simulink model "rlgrindingsystemPIDTune"  (R2024b)
settings: Solver=ode45  StartTime=0.0  StopTime=200  RelTol=1e-3  EnableMultiTasking=on
undefined symbols (not defined in the file or in its folder): DiscIntNeverNeededParam, Ts
libraries: rllib x1
settings Model: Creator=The MathWorks, Inc.  LastModifiedBy=phama
settings SolverCC: AlgebraicLoopSolver=TrustRegion  MaxZcPerStep=1
settings DataIOCC: LimitDataPoints=on  SaveFormat=Array  SignalLoggingName=logsOut
settings OptimizationCC: ExpressionDepthLimit=2147483647  InitFltsAndDblsToZero=on  LifeSpan=inf
settings DebuggingCC: SaveWithParameterizedLinksMsg=none  UnderspecifiedInitializationDetection=Classic  MergeDetectMultiDrivingBlocksExec=none  SignalResolutionControl=TryResolveAllWithWarning  MultiTaskDSMMsg=warning  FcnCallInpInsideContextMsg=warning  UnconnectedInputMsg=warning  UnconnectedOutputMsg=warning  UnconnectedLineMsg=warning  AllowSymbolicDim=off  StateNameClashWarn=warning  SFUnexpectedBacktrackingDiag=warning  SFNoUnconditionalDefaultTransitionDiag=warning  SFExecutionAtInitializationDiag=none  ArithmeticOperatorsInVariantConditions=warning
settings HardwareCC: ProdBitPerPointer=32  ProdBitPerSizeT=32  ProdBitPerPtrDiffT=32  ProdLargestAtomicFloat=None  ProdIntDivRoundTo=Undefined  ProdEndianess=Unspecified  ProdWordSize=32  ProdHWDeviceType=Specified
settings ModelReferenceCC: EnableRefExpFcnMdlSchedulingChecks=on  PropagateSignalLabelsOutOfModel=off
settings SFSimCC: SimUseLocalCustomCode=off
settings RTWCC: RTWUseLocalCustomCode=off  GPUComputeCapability=3.5  DLArmComputeVersion=19.05
settings CodeAppCC: StateflowObjectComments=on
settings GRTTargetCC: TargetFcnLib=ansi_tfl_tmw.mat  TargetLangStandard=C89/C90 (ANSI)  CombineOutputUpdateFcns=off  GRTInterface=on
settings ConfigComp: CovMetricSettings=dw  CovSaveCumulativeToWorkspaceVar=on  CovSaveSingleToWorkspaceVar=on  CovExternalEMLEnable=off

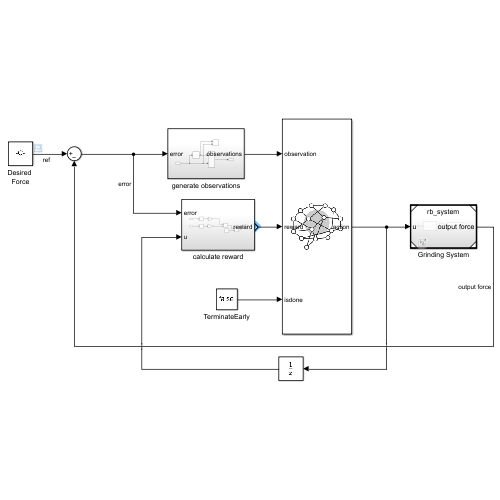
[thumbnail: Simulink's stored preview of the top-level diagram]
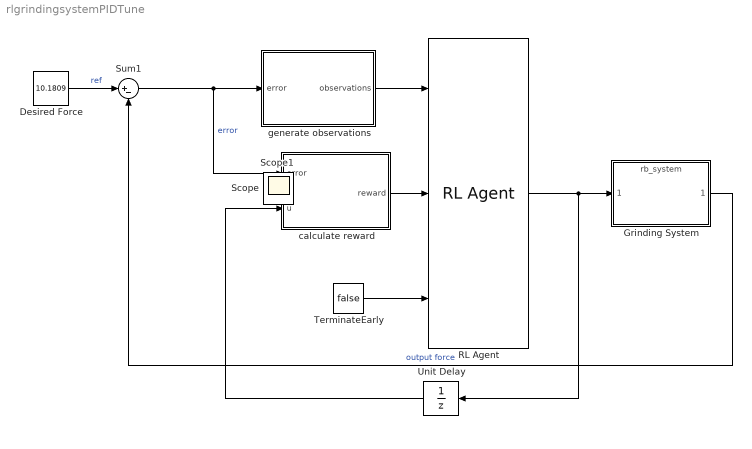
== system rlgrindingsystemPIDTune ==
  Desired Force : Constant  Value=10.1809
  Grinding System : ModelReference  ModelNameDialog=rb_system.slx  SimulationMode=Normal  ModelReferenceVersion=1.5
  RL Agent : rllib/RL Agent  Agent=agent  ExternalActionAsInput=off  ProvideLastAction=off  ProvideCumRwd=off  TreatAsDirectFeedthrough=on  UseStrictObservationDataTypes=off
  Sum1 : Sum  Inputs=|+-  SaturateOnIntegerOverflow=on
  TerminateEarly : Constant  Value=false
  Unit Delay : UnitDelay  SampleTime=-1  HasFrameUpgradeWarning=on
  calculate reward : Subsystem
  generate observations : Subsystem
  Scope : Scope
  Scope1 : Scope
  wires:
  Desired Force/1 -> Sum1/1  "ref"
  Sum1/1 -> calculate reward/1(error), generate observations/1(error)  "error"
  generate observations/1(observations) -> RL Agent/1
  RL Agent/1 -> Grinding System/1, Unit Delay/1
  Grinding System/1 -> Sum1/2  "output force"
  Unit Delay/1 -> calculate reward/2(u)
  calculate reward/1(reward) -> RL Agent/2
  TerminateEarly/1 -> RL Agent/3

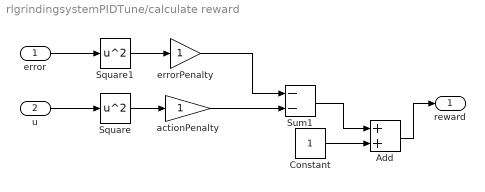
== system rlgrindingsystemPIDTune/calculate reward ==
  error : Inport
  u : Inport  Port=2
  Add : Sum
  Constant : Constant
  Square : Math  Operator=square
  Square1 : Math  Operator=square
  Sum1 : Sum  Inputs=--  OutDataTypeStr=double
  actionPenalty : Gain
  errorPenalty : Gain
  reward : Outport  VectorParamsAs1DForOutWhenUnconnected=off
  wires:
  Square1/1 -> errorPenalty/1
  errorPenalty/1 -> Sum1/1
  actionPenalty/1 -> Sum1/2
  Square/1 -> actionPenalty/1
  u/1 -> Square/1
  error/1 -> Square1/1
  Sum1/1 -> Add/1
  Add/1 -> reward/1
  Constant/1 -> Add/2

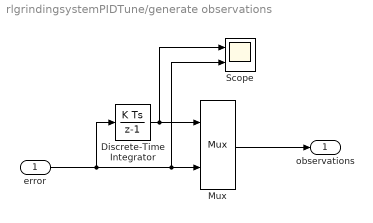
== system rlgrindingsystemPIDTune/generate observations ==
  error : Inport
  Discrete-Time Integrator : DiscreteIntegrator  SampleTime=Ts  ICPrevOutput=DiscIntNeverNeededParam  ICPrevScaledInput=DiscIntNeverNeededParam
  Mux : Mux  Inputs=2
  Scope : Scope  NumInputPorts=2
  observations : Outport  VectorParamsAs1DForOutWhenUnconnected=off
  wires:
  Discrete-Time Integrator/1 -> Scope/1, Mux/1
  error/1 -> Discrete-Time Integrator/1, Scope/2, Mux/2
  Mux/1 -> observations/1
